simulink model "Fuzzy_mf"  (R2014a)
settings: Solver=ode45  StartTime=0.0  StopTime=10.0  RelTol=1e-3
libraries: simulink x3
settings Model: Creator=w  LastModifiedBy=w

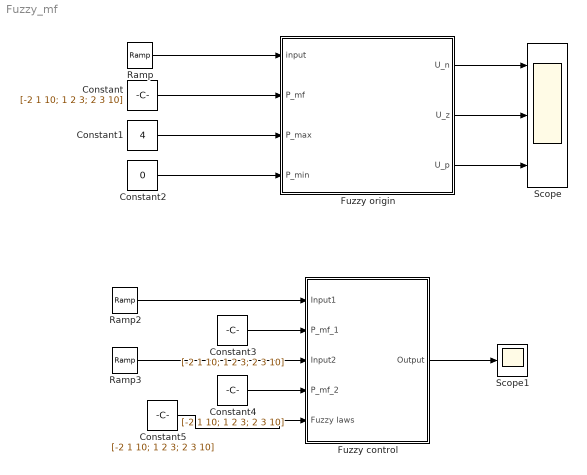
== system Fuzzy_mf ==
  Constant{,3..5} (4 alike) : Constant  Value=[-2 1 10; 1 2 3; 2 3 10]
  Constant1 : Constant  Value=4
  Constant2 : Constant  Value=0
  Fuzzy control : Subsystem
  Fuzzy origin : MATLAB Function  TreatAsAtomicUnit=on
  Ramp : simulink/Sources/Ramp  slope=1  start=0  X0=0
  Ramp2 : simulink/Sources/Ramp  slope=1  start=0  X0=0
  Ramp3 : simulink/Sources/Ramp  slope=1  start=0  X0=0
  Scope : Scope  NumInputPorts=3
      settings: YMin=-5~-5~-5  YMax=5~5~5
  Scope1 : Scope
  wires:
  Fuzzy origin/1(U_n) -> Scope/1
  Fuzzy origin/2(U_z) -> Scope/2
  Fuzzy origin/3(U_p) -> Scope/3
  Ramp/1 -> Fuzzy origin/1(input)
  Constant/1 -> Fuzzy origin/2(P_mf)
  Constant1/1 -> Fuzzy origin/3(P_max)
  Constant2/1 -> Fuzzy origin/4(P_min)
  Constant3/1 -> Fuzzy control/2(P_mf_1)
  Constant4/1 -> Fuzzy control/4(P_mf_2)
  Ramp2/1 -> Fuzzy control/1(Input1)
  Ramp3/1 -> Fuzzy control/3(Input2)
  Constant5/1 -> Fuzzy control/5(Fuzzy laws)
  Fuzzy control/1(Output) -> Scope1/1

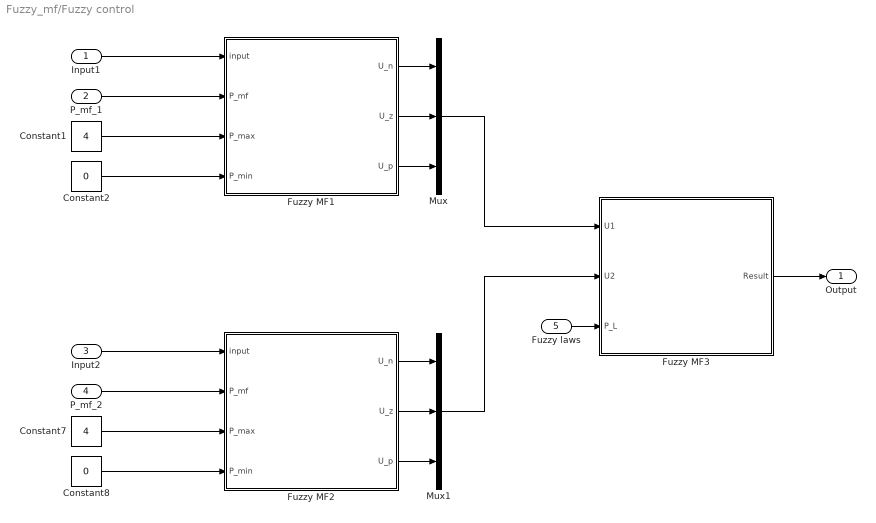
== system Fuzzy_mf/Fuzzy control ==
  Input1 : Inport
  P_mf_1 : Inport  Port=2
  Input2 : Inport  Port=3
  P_mf_2 : Inport  Port=4
  Fuzzy laws : Inport  Port=5
  Constant1 : Constant  Value=4
  Constant2 : Constant  Value=0
  Constant7 : Constant  Value=4
  Constant8 : Constant  Value=0
  Fuzzy MF1 : MATLAB Function  TreatAsAtomicUnit=on
  Fuzzy MF2 : MATLAB Function  TreatAsAtomicUnit=on
  Fuzzy MF3 : MATLAB Function  TreatAsAtomicUnit=on
  Mux : Mux  Inputs=3
  Mux1 : Mux  Inputs=3
  Output : Outport
  wires:
  Fuzzy MF2/2(U_z) -> Mux1/2
  Fuzzy MF1/3(U_p) -> Mux/3
  Fuzzy MF1/1(U_n) -> Mux/1
  Fuzzy MF1/2(U_z) -> Mux/2
  Mux/1 -> Fuzzy MF3/1(U1)
  Mux1/1 -> Fuzzy MF3/2(U2)
  P_mf_1/1 -> Fuzzy MF1/2(P_mf)
  Constant1/1 -> Fuzzy MF1/3(P_max)
  Constant2/1 -> Fuzzy MF1/4(P_min)
  Fuzzy MF2/1(U_n) -> Mux1/1
  Fuzzy MF2/3(U_p) -> Mux1/3
  Fuzzy laws/1 -> Fuzzy MF3/3(P_L)
  Input2/1 -> Fuzzy MF2/1(input)
  Constant8/1 -> Fuzzy MF2/4(P_min)
  Constant7/1 -> Fuzzy MF2/3(P_max)
  P_mf_2/1 -> Fuzzy MF2/2(P_mf)
  Fuzzy MF3/1(Result) -> Output/1
  Input1/1 -> Fuzzy MF1/1(input)

== matlab function Fuzzy_mf/Fuzzy control/Fuzzy MF1 ==
  data: input input; U_n output; U_z output; U_p output; P_mf input; P_max input; P_min input
function [U_n,U_z,U_p] = Fuzzy_mf(input,P_mf,P_max,P_min)
% This is a function to fuzzy the input varriables, there are 3mf in one
% module.
%% check & modify the elements in the parameters matrix
U_n=0;U_z=0;U_p=0;
P_mf(1,1)=P_min;
P_mf(3,3)=P_max;
% a>=P_min & c<P_max
for i=1:3
    if P_mf(i,1)<P_min
        P_mf(i,1)=P_min;
    end
    if P_mf(i,3)>P_max
        P_mf(i,3)=P_max;
    end
end
% a<c, a<b<c
for i=1:3
    if P_mf(i,3)<=P_mf(i,1)
       P_mf(i,3)=P_mf(i,1)+0.1; 
    end
    if P_mf(i,2)<=P_mf(i,1)
       P_mf(i,2)=P_mf(i,1)+0.05; 
    end
    if P_mf(i,3)<=P_mf(i,2)
       P_mf(i,2)=P_mf(i,3)-0.05; 
    end
end
% xn<xz<xp
for j=1:3
    if P_mf(3,j)<=P_mf(1,j)
       P_mf(3,j)=P_mf(1,j)+0.1; 
    end
    if P_mf(2,j)<=P_mf(1,j)
       P_mf(2,j)=P_mf(1,j)+0.05; 
    end
    if P_mf(3,j)<=P_mf(2,j)
       P_mf(2,j)=P_mf(1,j)-0.05; 
    end
end
%% caulate the membership value
% for U_n
tmp=1;
for i=1:3
    if input<=P_mf(i,1)||input>=P_mf(i,3)
        tmp=0;
    end
    if input>P_mf(i,1)&&input<=P_mf(i,2)
        tmp=(input-P_mf(i,1))/(P_mf(i,2)-P_mf(i,1));
    end
    if input>P_mf(i,2)&&input<P_mf(i,3)
        tmp=(input-P_mf(i,3))/(P_mf(i,2)-P_mf(i,3));
    end
    if i==1
        U_n=tmp;
    end
    if i==2
        U_z=tmp;
    end
    if i==3
        U_p=tmp;
    end
end

== matlab function Fuzzy_mf/Fuzzy origin ==
  data: input input; U_n output; U_z output; U_p output; P_mf input; P_max input; P_min input
function [U_n,U_z,U_p] = Fuzzy_mf(input,P_mf,P_max,P_min)
% This is a function to fuzzy the input varriables, there are 3mf in one
% module.
%% check & modify the elements in the parameters matrix
U_n=0;U_z=0;U_p=0;
P_mf(1,1)=P_min;
P_mf(3,3)=P_max;
% a>=P_min & c<P_max
for i=1:3
    if P_mf(i,1)<P_min
        P_mf(i,1)=P_min;
    end
    if P_mf(i,3)>P_max
        P_mf(i,3)=P_max;
    end
end
% a<c, a<b<c
for i=1:3
    if P_mf(i,3)<=P_mf(i,1)
       P_mf(i,3)=P_mf(i,1)+0.1; 
    end
    if P_mf(i,2)<=P_mf(i,1)
       P_mf(i,2)=P_mf(i,1)+0.05; 
    end
    if P_mf(i,3)<=P_mf(i,2)
       P_mf(i,2)=P_mf(i,3)-0.05; 
    end
end
% xn<xz<xp
for j=1:3
    if P_mf(3,j)<=P_mf(1,j)
       P_mf(3,j)=P_mf(1,j)+0.1; 
    end
    if P_mf(2,j)<=P_mf(1,j)
       P_mf(2,j)=P_mf(1,j)+0.05; 
    end
    if P_mf(3,j)<=P_mf(2,j)
       P_mf(2,j)=P_mf(1,j)-0.05; 
    end
end
%% caulate the membership value
% for U_n
tmp=1;
for i=1:3
    if input<=P_mf(i,1)||input>=P_mf(i,3)
        tmp=0;
    end
    if input>P_mf(i,1)&&input<=P_mf(i,2)
        tmp=(input-P_mf(i,1))/(P_mf(i,2)-P_mf(i,1));
    end
    if input>P_mf(i,2)&&input<P_mf(i,3)
        tmp=(input-P_mf(i,3))/(P_mf(i,2)-P_mf(i,3));
    end
    if i==1
        U_n=tmp;
    end
    if i==2
        U_z=tmp;
    end
    if i==3
        U_p=tmp;
    end
end

== matlab function Fuzzy_mf/Fuzzy control/Fuzzy MF2 ==
  data: input input; U_n output; U_z output; U_p output; P_mf input; P_max input; P_min input
function [U_n,U_z,U_p] = Fuzzy_mf(input,P_mf,P_max,P_min)
% This is a function to fuzzy the input varriables, there are 3mf in one
% module.
%% check & modify the elements in the parameters matrix
U_n=0;U_z=0;U_p=0;
P_mf(1,1)=P_min;
P_mf(3,3)=P_max;
% a>=P_min & c<P_max
for i=1:3
    if P_mf(i,1)<P_min
        P_mf(i,1)=P_min;
    end
    if P_mf(i,3)>P_max
        P_mf(i,3)=P_max;
    end
end
% a<c, a<b<c
for i=1:3
    if P_mf(i,3)<=P_mf(i,1)
       P_mf(i,3)=P_mf(i,1)+0.1; 
    end
    if P_mf(i,2)<=P_mf(i,1)
       P_mf(i,2)=P_mf(i,1)+0.05; 
    end
    if P_mf(i,3)<=P_mf(i,2)
       P_mf(i,2)=P_mf(i,3)-0.05; 
    end
end
% xn<xz<xp
for j=1:3
    if P_mf(3,j)<=P_mf(1,j)
       P_mf(3,j)=P_mf(1,j)+0.1; 
    end
    if P_mf(2,j)<=P_mf(1,j)
       P_mf(2,j)=P_mf(1,j)+0.05; 
    end
    if P_mf(3,j)<=P_mf(2,j)
       P_mf(2,j)=P_mf(1,j)-0.05; 
    end
end
%% caulate the membership value
% for U_n
tmp=1;
for i=1:3
    if input<=P_mf(i,1)||input>=P_mf(i,3)
        tmp=0;
    end
    if input>P_mf(i,1)&&input<=P_mf(i,2)
        tmp=(input-P_mf(i,1))/(P_mf(i,2)-P_mf(i,1));
    end
    if input>P_mf(i,2)&&input<P_mf(i,3)
        tmp=(input-P_mf(i,3))/(P_mf(i,2)-P_mf(i,3));
    end
    if i==1
        U_n=tmp;
    end
    if i==2
        U_z=tmp;
    end
    if i==3
        U_p=tmp;
    end
end

== matlab function Fuzzy_mf/Fuzzy control/Fuzzy MF3 ==
  data: U1 input; Result output; U2 input; P_L input
function Result  = Defuzz(U1,U2,P_L)
% 0 order of TS, weight average method
%% caculate the weight of each rule 
w=zeros(3,3);
Result=0;
for i=1:3
    for j=1:3
        w(i,j)=U1(i)*U2(j);
    end
end
w_sum=sum(sum(w));
%% weight average method for the output 
for i=1:3
    for j=1:3
        Result=Result+w(i,j)/w_sum*P_L(i,j);
    end
end
